simulink model "doublePendulumIMU"  (R2024b)
settings: Solver=VariableStepAuto  StartTime=0.0  StopTime=10.0  MaxStep=0.01  RelTol=1e-3  AbsTol=1e-3  EnableMultiTasking=on
undefined symbols (not defined in the file or in its folder): fractalcoef, X, Y, Z
libraries: nesl_utility x27, sm_lib x11, mspsensorlib x8, matrix_library x2
settings Model: DataDictionary=simData.sldd  Creator=The MathWorks, Inc.  LastModifiedBy=jfing
settings SolverCC: AutoScaleAbsTol=off  AlgebraicLoopSolver=TrustRegion  MaxZcPerStep=1
settings DataIOCC: LimitDataPoints=on  MaxDataPoints=10000
settings OptimizationCC: ReuseModelBlockBuffer=off  LifeSpan=inf
settings DebuggingCC: UnconnectedInputMsg=warning  UnconnectedOutputMsg=warning  UnconnectedLineMsg=warning  AllowSymbolicDim=off  SFUnexpectedBacktrackingDiag=warning  SFNoUnconditionalDefaultTransitionDiag=warning  SFExecutionAtInitializationDiag=none  ArithmeticOperatorsInVariantConditions=warning
settings HardwareCC: ProdHWDeviceType=AMD->x86-64 (Windows64)
settings ModelReferenceCC: EnableRefExpFcnMdlSchedulingChecks=on  EnableParallelModelReferenceBuilds=on  ParallelModelReferenceMATLABWorkerInit=Load Top Model
settings SFSimCC: SimUseLocalCustomCode=off  UsePrecompiledLibraries=Avoid  CustomCodeUndefinedFunction=UseInterfaceOnly  SimTargetLang=C++  GPUAcceleration=on  SimGPUMallocThreshold=1000  SimGPUStackLimitPerThread=2048  SimDLTargetLibrary=cudnn
settings RTWCC: RTWUseLocalCustomCode=off  GPUComputeCapability=3.5  DLArmComputeVersion=19.05
settings CodeAppCC: StateflowObjectComments=on
settings GRTTargetCC: TargetLangStandard=C89/C90 (ANSI)
settings ConfigComp: CovMetricSettings=dw  CovSaveCumulativeToWorkspaceVar=on  CovSaveSingleToWorkspaceVar=on  CovExternalEMLEnable=off  CovSFcnEnable=off
settings SimscapeCC: SimscapeLogType=all  SimscapeLogSimulationStatistics=on  SimscapeLogDataHistory=10000

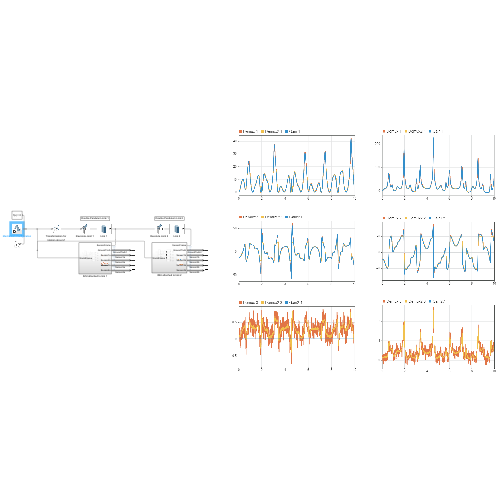
[thumbnail: Simulink's stored preview of the top-level diagram]
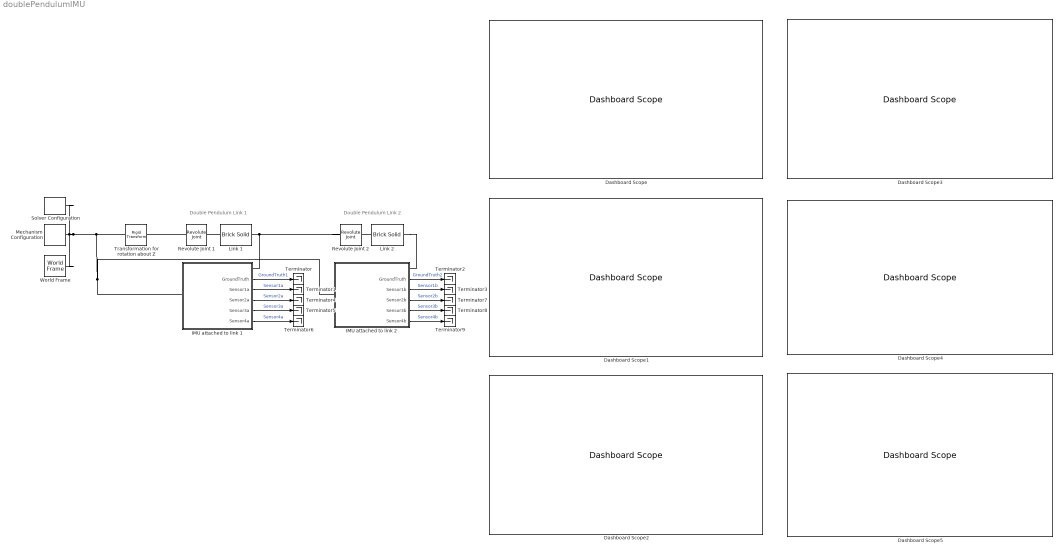
== system doublePendulumIMU ==
  note: Double Pendulum Link 1
  note: Double Pendulum Link 2
  Dashboard Scope{,1..5} (6 alike) : DashboardScope
  IMU attached to link 1 : Subsystem
      settings: PortSchema="{\"entries\":[{\"content\":{\"sides\":[{\"content\":{},\"type\":\"ConnectorPlacement.EquallySpacedRectSide\",\"uuid\":\"7a848249-f78c-431e-84de-981fe01eaf41\"},{\"content\":{\"side\":\"RIGHT\"},\"type\":\"ConnectorPlacement.EquallySpacedRectSide\",\"uuid\":\"a7aca224-ae93-4c7d-a6de-e3d97876bf59\"},{\"content\":{\"connectorIds\":[\"LConn1\"],\"side\":\"TOP\"},\"type\":\"ConnectorPlacement.EquallySpacedRectSide\",\"uuid\":\"e9c2225b-3f07-428c-8b88-abfc95f79ce3\"},{\"content\":{\"connectorIds\":[\"RConn1\",\"Out1\",\"Out2\",\"Out3\",\"Out4\",\"Out5\"],\"side\":\"BOTTOM\"},\"type\":\"ConnectorPlacement.EquallySpacedRectSide\",\"uuid\":\"5c87de37-5620-4b71-be74-049ce4a9ec5b\"}]},\"type\":\"ConnectorPlacement.EquallySpacedConnector\",\"uuid\":\"7bd4f58a-19d1-4168-9367-fe9ef4865104\"}],\"packageUris\":[\"http://schema.mathworks.com/mf0/Connector/R2020b\"],\"version\":\"1.0\"}"
  IMU attached to link 2 : Subsystem
      settings: PortSchema="{\"entries\":[{\"content\":{\"sides\":[{\"content\":{},\"type\":\"ConnectorPlacement.EquallySpacedRectSide\",\"uuid\":\"7a848249-f78c-431e-84de-981fe01eaf41\"},{\"content\":{\"side\":\"RIGHT\"},\"type\":\"ConnectorPlacement.EquallySpacedRectSide\",\"uuid\":\"a7aca224-ae93-4c7d-a6de-e3d97876bf59\"},{\"content\":{\"connectorIds\":[\"LConn1\"],\"side\":\"TOP\"},\"type\":\"ConnectorPlacement.EquallySpacedRectSide\",\"uuid\":\"e9c2225b-3f07-428c-8b88-abfc95f79ce3\"},{\"content\":{\"connectorIds\":[\"RConn1\",\"Out1\",\"Out2\",\"Out3\",\"Out4\",\"Out5\"],\"side\":\"BOTTOM\"},\"type\":\"ConnectorPlacement.EquallySpacedRectSide\",\"uuid\":\"5c87de37-5620-4b71-be74-049ce4a9ec5b\"}]},\"type\":\"ConnectorPlacement.EquallySpacedConnector\",\"uuid\":\"7bd4f58a-19d1-4168-9367-fe9ef4865104\"}],\"packageUris\":[\"http://schema.mathworks.com/mf0/Connector/R2020b\"],\"version\":\"1.0\"}"
  Link 1 : sm_lib/Body Elements/Brick Solid  BrickDimensions=[1 0.1 0.1]  BrickDimensionsUnits=m  ExportEntireGeometry=off  InertiaType=CalculateFromGeometry  BasedOnType=Density  Density=1000  DensityUnits=kg/m^3  Mass=1  MassUnits=kg  CenterOfMass=[0 0 0]  CenterOfMassUnits=m  MomentsOfInertia=[1 1 1]  MomentsOfInertiaUnits=kg*m^2  ProductsOfInertia=[0 0 0]  ProductsOfInertiaUnits=kg*m^2  GraphicType=FromGeometry  MarkerShape=Sphere  MarkerSize=10  GraphicVisPropType=SimpleVisualProperties  GraphicDiffuseColor=[0.5 0.5 0.5]  GraphicOpacity=1.0  GraphicSpecularColor=[0.5 0.5 0.5 1.0]  GraphicAmbientColor=[0.15 0.15 0.15 1.0]  GraphicEmissiveColor=[0.0 0.0 0.0 1.0]  GraphicShininess=75  DoExposeReferenceFrame=off  SerializedFrames=<Frames><Frame><Id>Frame1</Id><Value><Name>F1</Name><Origin><Source>GeometricFeature</Source><FeatureName>-x surface</FeatureName></Origin><PrimaryAxis><DefinedDirection>+Z</DefinedDirection><Source>ReferenceFrame</Source><SourceDirection>+Z</SourceDirection><FeatureName></FeatureName></PrimaryAxis><SecondaryAxis><DefinedDirection>+X</DefinedDirection><Source>ReferenceFrame</Source><SourceDirection>+X</SourceDirection><FeatureName></FeatureName></SecondaryAxis></Value></Frame><Frame><Id>Frame2</Id><Value><Name>F2</Name><Origin><Source>GeometricFeature</Source><FeatureName>+x surface</FeatureName></Origin><PrimaryAxis><DefinedDirection>+Z</DefinedDirection><Source>ReferenceFrame</Source><SourceDirection>+Z</SourceDirection><FeatureName></FeatureName></PrimaryAxis><SecondaryAxis><DefinedDirection>+X</DefinedDirection><Source>ReferenceFrame</Source><SourceDirection>+X</SourceDirection><FeatureName></FeatureName></SecondaryAxis></Value></Frame></Frames>
  Link 2 : sm_lib/Body Elements/Brick Solid  BrickDimensions=[1 0.1 0.1]  BrickDimensionsUnits=m  ExportEntireGeometry=off  InertiaType=CalculateFromGeometry  BasedOnType=Density  Density=1000  DensityUnits=kg/m^3  Mass=1  MassUnits=kg  CenterOfMass=[0 0 0]  CenterOfMassUnits=m  MomentsOfInertia=[1 1 1]  MomentsOfInertiaUnits=kg*m^2  ProductsOfInertia=[0 0 0]  ProductsOfInertiaUnits=kg*m^2  GraphicType=FromGeometry  MarkerShape=Sphere  MarkerSize=10  GraphicVisPropType=SimpleVisualProperties  GraphicDiffuseColor=[0.5 0.5 0.5]  GraphicOpacity=1.0  GraphicSpecularColor=[0.5 0.5 0.5 1.0]  GraphicAmbientColor=[0.15 0.15 0.15 1.0]  GraphicEmissiveColor=[0.0 0.0 0.0 1.0]  GraphicShininess=75  DoExposeReferenceFrame=off  SerializedFrames=<Frames><Frame><Id>Frame1</Id><Value><Name>F1</Name><Origin><Source>GeometricFeature</Source><FeatureName>-x surface</FeatureName></Origin><PrimaryAxis><DefinedDirection>+Z</DefinedDirection><Source>ReferenceFrame</Source><SourceDirection>+Z</SourceDirection><FeatureName></FeatureName></PrimaryAxis><SecondaryAxis><DefinedDirection>+X</DefinedDirection><Source>ReferenceFrame</Source><SourceDirection>+X</SourceDirection><FeatureName></FeatureName></SecondaryAxis></Value></Frame><Frame><Id>Frame2</Id><Value><Name>F2</Name><Origin><Source>GeometricFeature</Source><FeatureName>+x surface</FeatureName></Origin><PrimaryAxis><DefinedDirection>+Z</DefinedDirection><Source>ReferenceFrame</Source><SourceDirection>+Z</SourceDirection><FeatureName></FeatureName></PrimaryAxis><SecondaryAxis><DefinedDirection>+X</DefinedDirection><Source>ReferenceFrame</Source><SourceDirection>+X</SourceDirection><FeatureName></FeatureName></SecondaryAxis></Value></Frame></Frames>
  Mechanism Configuration : sm_lib/Utilities/Mechanism Configuration  UniformGravity=Constant  GravityVector=[0 0 -9.80665]  GravityVectorUnits=m/s^2  LinearizationDelta=0.001  JointModeTransitionNonlinearIterations=2
  Revolute Joint 1 : sm_lib/Joints/Revolute Joint  JointMode=Normal  CompositeWrenchDir=FollowerOnBase  CompositeWrenchFrame=BaseFrame  SenseConstraintForce=off  SenseConstraintTorque=off  SenseTotalForce=off  SenseTotalTorque=off  PositionTargetSpecify=off  PositionTargetPriority=High  PositionTargetValue=0  PositionTargetValueUnits=deg  VelocityTargetSpecify=off  VelocityTargetPriority=High  VelocityTargetValue=0  VelocityTargetValueUnits=deg/s  EquilibriumPosition=0  EquilibriumPositionUnits=deg  SpringStiffness=0  SpringStiffnessUnits=N*m/deg  DampingCoefficient=0  DampingCoefficientUnits=N*m/(deg/s)  LowerLimitSpecify=off  LowerLimitBound=-90  LowerLimitBoundUnits=deg  LowerLimitStiffness=1e4  LowerLimitStiffnessUnits=N*m/deg  LowerLimitDamping=10  LowerLimitDampingUnits=N*m/(deg/s)  LowerLimitTransitionRegionWidth=0.1  LowerLimitTransitionRegionWidthUnits=deg  UpperLimitSpecify=off  UpperLimitBound=90  UpperLimitBoundUnits=deg  UpperLimitStiffness=1e4  UpperLimitStiffnessUnits=N*m/deg  UpperLimitDamping=10  UpperLimitDampingUnits=N*m/(deg/s)  UpperLimitTransitionRegionWidth=0.1  UpperLimitTransitionRegionWidthUnits=deg  TorqueActuationMode=NoTorque  MotionActuationMode=ComputedMotion  SensePosition=off  SenseVelocity=off  SenseAcceleration=off  SenseTorqueForce=off  SenseLowerLimitTorqueForce=off  SenseUpperLimitTorqueForce=off
  Revolute Joint 2 : sm_lib/Joints/Revolute Joint  JointMode=Normal  CompositeWrenchDir=FollowerOnBase  CompositeWrenchFrame=BaseFrame  SenseConstraintForce=off  SenseConstraintTorque=off  SenseTotalForce=off  SenseTotalTorque=off  PositionTargetSpecify=off  PositionTargetPriority=High  PositionTargetValue=0  PositionTargetValueUnits=deg  VelocityTargetSpecify=off  VelocityTargetPriority=High  VelocityTargetValue=0  VelocityTargetValueUnits=deg/s  EquilibriumPosition=0  EquilibriumPositionUnits=deg  SpringStiffness=0  SpringStiffnessUnits=N*m/deg  DampingCoefficient=0  DampingCoefficientUnits=N*m/(deg/s)  LowerLimitSpecify=off  LowerLimitBound=-90  LowerLimitBoundUnits=deg  LowerLimitStiffness=1e4  LowerLimitStiffnessUnits=N*m/deg  LowerLimitDamping=10  LowerLimitDampingUnits=N*m/(deg/s)  LowerLimitTransitionRegionWidth=0.1  LowerLimitTransitionRegionWidthUnits=deg  UpperLimitSpecify=off  UpperLimitBound=90  UpperLimitBoundUnits=deg  UpperLimitStiffness=1e4  UpperLimitStiffnessUnits=N*m/deg  UpperLimitDamping=10  UpperLimitDampingUnits=N*m/(deg/s)  UpperLimitTransitionRegionWidth=0.1  UpperLimitTransitionRegionWidthUnits=deg  TorqueActuationMode=NoTorque  MotionActuationMode=ComputedMotion  SensePosition=off  SenseVelocity=off  SenseAcceleration=off  SenseTorqueForce=off  SenseLowerLimitTorqueForce=off  SenseUpperLimitTorqueForce=off
  Solver Configuration : nesl_utility/Solver Configuration  PhysicalDomain=network_engine_domain  SubClassName=solver  LeftPortType=input  RightPortType=generic  Tones=[]  Harmonics=[]  SimulateNoise=off  Profile=off  UseLocalSampling=off  EnableSwitchedLinearOptims=on  FrequencyDomain=off  UseCCode=off  RelTol=0.001  AbsTol=1e-06  MinStep=1e-09  ToWorkspace=off  RevertToSquareIcSolve=off  NumHomotopyIterations=100  PhasorMode=off  PhasorModeNumHarmonics=1  ConsistencySolver=NEWTON_XTOL_AFTER_FTOL  IndexReductionMethod=DerivativeReplacement  DoDC=off  ResidualTolerance=1e-09  ConsistencyTolSource=GLOBAL  ConsistencyAbsTol=0.001  ConsistencyRelTol=0.001  ConsistencyTolFactor=0.001  UseLocalSolver=off  LocalSolverChoice=NE_BACKWARD_EULER_ADVANCER  ResolveIndetEquations=on  FunctionEvalNumThread=1  LocalSolverSampleTime=0.001  DoFixedCost=off  MaxNonlinIter=3  MaxModeIter=2  ComputeImpulses=off  ImpulseIterations=2  LinearAlgebra=Sparse  LinearAlgebraNumThread=0  EquationFormulation=NE_TIME_EF  DelaysMemoryBudget=1024  AutomaticFiltering=on  FilteringTimeConstant=0.001  PartitionStorageMethod=AS_NEEDED  PartitionMemoryBudget=1024  PartitionMethod=FAST  MultibodyUseLocalSolver=off  MultibodyLocalSolverChoice=ODE1  MultibodyLocalSolverSampleTime=0.001
  Terminator{,1..9} (10 alike) : Terminator
  Transformation for rotation about Z : sm_lib/Frames and Transforms/Rigid Transform  RotationMethod=StandardAxis  FollAlignAxisA=+X  BaseAlignAxisA=+Y  FollAlignAxisB=+Y  BaseAlignAxisB=+Z  RotationStandardAxis=-X  RotationAngle=90  RotationAngleUnits=deg  RotationArbitraryAxis=[0 0 1]  RotationSequenceAxes=FollowerAxes  RotationSequence=XYX  RotationSequenceAngles=[0 0 0]  RotationSequenceAnglesUnits=deg  RotationMatrix=[1 0 0; 0 1 0; 0 0 1]  Quaternion=[1 0 0 0]  TranslationMethod=None  TranslationCartesianOffset=[0 0 0]  TranslationCartesianOffsetUnits=m  TranslationStandardAxis=+Z  TranslationStandardOffset=0  TranslationStandardOffsetUnits=m  TranslationROffset=0  TranslationROffsetUnits=m  TranslationThetaOffset=0  TranslationThetaOffsetUnits=deg  TranslationZOffset=0  TranslationZOffsetUnits=m
  World Frame : sm_lib/Frames and Transforms/World Frame
  wires:
  IMU attached to link 1/1(GroundTruth) -> Terminator/1  "GroundTruth1"
  IMU attached to link 1/2(Sensor1a) -> Terminator1/1  "Sensor1a"
  IMU attached to link 2/2(Sensor1b) -> Terminator3/1  "Sensor1b"
  IMU attached to link 2/1(GroundTruth) -> Terminator2/1  "GroundTruth2"
  IMU attached to link 1/3(Sensor2a) -> Terminator4/1  "Sensor2a"
  IMU attached to link 1/4(Sensor3a) -> Terminator5/1  "Sensor3a"
  IMU attached to link 1/5(Sensor4a) -> Terminator6/1  "Sensor4a"
  IMU attached to link 2/3(Sensor2b) -> Terminator7/1  "Sensor2b"
  IMU attached to link 2/4(Sensor3b) -> Terminator8/1  "Sensor3b"
  IMU attached to link 2/5(Sensor4b) -> Terminator9/1  "Sensor4b"
  connections:
  Link 1/LConn1 -- Revolute Joint 1/RConn1
  Revolute Joint 1/LConn1 -- Transformation for rotation about Z/RConn1
  IMU attached to link 1/RConn1 -- Revolute Joint 2/LConn1 -- Link 1/RConn1
  Link 2/LConn1 -- Revolute Joint 2/RConn1
  Link 2/RConn1 -- IMU attached to link 2/RConn1
  IMU attached to link 1/LConn1 -- IMU attached to link 2/LConn1 -- Transformation for rotation about Z/LConn1 -- World Frame/RConn1 -- Solver Configuration/RConn1 -- Mechanism Configuration/RConn1

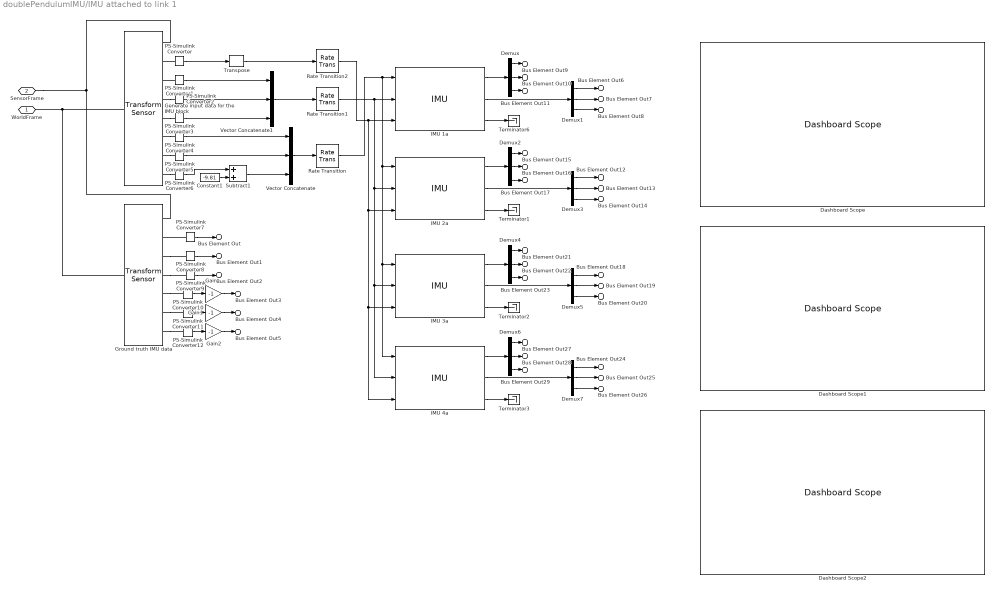
== system doublePendulumIMU/IMU attached to link 1 ==
  Constant1 : Constant  Value=-9.81
  Dashboard Scope : DashboardScope
  Dashboard Scope1 : DashboardScope
  Dashboard Scope2 : DashboardScope
  Demux{,1..7} (8 alike) : Demux  Outputs=3
  Gain : Gain  Gain=-1
  Gain1 : Gain  Gain=-1
  Gain2 : Gain  Gain=-1
  Generate input data for the IMU block : sm_lib/Frames and Transforms/Transform Sensor  MeasurementFrame=World  RotationSequence=XYX  SenseAngle=off  SenseAxis=off  SenseQ=on  SenseR=off  SenseRotationSequence=off  SenseOmegaX=on  SenseOmegaY=on  SenseOmegaZ=on  SenseOmega=off  SenseQDot=off  SenseRDot=off  SenseRotationSequenceDot=off  SenseAlphaX=off  SenseAlphaY=off  SenseAlphaZ=off  SenseAlpha=off  SenseQDDot=off  SenseRDDot=off  SenseX=off  SenseY=off  SenseZ=off  SenseXYZ=off  SenseRad=off  SenseAzim=off  SenseDist=off  SenseInc=off  SenseXDot=off  SenseYDot=off  SenseZDot=off  SenseXYZDot=off  SenseRadDot=off  SenseAzimDot=off  SenseDistDot=off  SenseIncDot=off  SenseXDDot=on  SenseYDDot=on  SenseZDDot=on  SenseXYZDDot=off  SenseRadDDot=off  SenseAzimDDot=off  SenseDistDDot=off  SenseIncDDot=off
  Ground truth IMU data : sm_lib/Frames and Transforms/Transform Sensor  MeasurementFrame=NonRotatingFollower  RotationSequence=XYX  SenseAngle=off  SenseAxis=off  SenseQ=off  SenseR=off  SenseRotationSequence=off  SenseOmegaX=on  SenseOmegaY=on  SenseOmegaZ=on  SenseOmega=off  SenseQDot=off  SenseRDot=off  SenseRotationSequenceDot=off  SenseAlphaX=off  SenseAlphaY=off  SenseAlphaZ=off  SenseAlpha=off  SenseQDDot=off  SenseRDDot=off  SenseX=off  SenseY=off  SenseZ=off  SenseXYZ=off  SenseRad=off  SenseAzim=off  SenseDist=off  SenseInc=off  SenseXDot=off  SenseYDot=off  SenseZDot=off  SenseXYZDot=off  SenseRadDot=off  SenseAzimDot=off  SenseDistDot=off  SenseIncDot=off  SenseXDDot=on  SenseYDDot=on  SenseZDDot=on  SenseXYZDDot=off  SenseRadDDot=off  SenseAzimDDot=off  SenseDistDDot=off  SenseIncDDot=off
  IMU 1a : mspsensorlib/IMU  DispRefFrame=ENU  TemperaturePort=off  Temperature=25  MagneticFieldPort=off  MagneticFieldNED=[ 27.5550, -2.4169, -16.0849 ]  MagneticFieldENU=[ -2.4169, 27.5550, 16.0849 ]  SeedDouble=67  SimulateUsing=Interpreted execution  AccelParamsMeasurementRange=156.9064  AccelParamsResolution=4.9791e-05  AccelParamsConstantBias=0.196133  AccelParamsAxesMisalignment=1  AccelParamsNoiseDensity=0.00063743225  AccelParamsBiasInstability=0.15691  AccelParamsBiasInstabilityNumerator=fractalcoef().Numerator  AccelParamsBiasInstabilityDenominator=fractalcoef().Denominator  AccelParamsRandomWalk=[ 0, 0, 0 ]  AccelParamsNoiseType=double-sided  AccelParamsTemperatureBias=0.0014709975  AccelParamsTemperatureScaleFactor=0.005  GyroParamsMeasurementRange=34.9066  GyroParamsResolution=3.4936  GyroParamsConstantBias=0.00872664625997165  GyroParamsAxesMisalignment=1.25  GyroParamsAccelerationBias=[ 0, 0, 0 ]  GyroParamsNoiseDensity=0.000488692190558412  GyroParamsBiasInstability=0.034907  GyroParamsBiasInstabilityNumerator=fractalcoef().Numerator  GyroParamsBiasInstabilityDenominator=fractalcoef().Denominator  GyroParamsRandomWalk=[ 0, 0, 0 ]  GyroParamsNoiseType=double-sided  GyroParamsTemperatureBias=8.72664625997165e-05  GyroParamsTemperatureScaleFactor=0.005  MagParamsMeasurementRange=Inf  MagParamsResolution=0  MagParamsConstantBias=[ 0, 0, 0 ]  MagParamsAxesMisalignment=[ 100, 0, 0; 0, 100, 0; 0, 0, 100 ]  MagParamsNoiseDensity=[ 0, 0, 0 ]  MagParamsBiasInstability=[ 0, 0, 0 ]  MagParamsBiasInstabilityNumerator=fractalcoef().Numerator  MagParamsBiasInstabilityDenominator=fractalcoef().Denominator  MagParamsRandomWalk=[ 0, 0, 0 ]  MagParamsNoiseType=double-sided  MagParamsTemperatureBias=[ 0, 0, 0 ]  MagParamsTemperatureScaleFactor=[ 0, 0, 0 ]
  IMU 2a : mspsensorlib/IMU  DispRefFrame=ENU  TemperaturePort=off  Temperature=25  MagneticFieldPort=off  MagneticFieldNED=[ 27.5550, -2.4169, -16.0849 ]  MagneticFieldENU=[ -2.4169, 27.5550, 16.0849 ]  SeedDouble=67  SimulateUsing=Interpreted execution  AccelParamsMeasurementRange=19.6133  AccelParamsResolution=6.2239e-06  AccelParamsConstantBias=0.196133  AccelParamsAxesMisalignment=1  AccelParamsNoiseDensity=0.00063743225  AccelParamsBiasInstability=0.019613  AccelParamsBiasInstabilityNumerator=fractalcoef().Numerator  AccelParamsBiasInstabilityDenominator=fractalcoef().Denominator  AccelParamsRandomWalk=[ 0, 0, 0 ]  AccelParamsNoiseType=double-sided  AccelParamsTemperatureBias=0.0014709975  AccelParamsTemperatureScaleFactor=0.005  GyroParamsMeasurementRange=4.3633  GyroParamsResolution=0.43737  GyroParamsConstantBias=0.00872664625997165  GyroParamsAxesMisalignment=1.25  GyroParamsAccelerationBias=[ 0, 0, 0 ]  GyroParamsNoiseDensity=0.000488692190558412  GyroParamsBiasInstability=0.0043633  GyroParamsBiasInstabilityNumerator=fractalcoef().Numerator  GyroParamsBiasInstabilityDenominator=fractalcoef().Denominator  GyroParamsRandomWalk=[ 0, 0, 0 ]  GyroParamsNoiseType=double-sided  GyroParamsTemperatureBias=8.72664625997165e-05  GyroParamsTemperatureScaleFactor=0.005  MagParamsMeasurementRange=Inf  MagParamsResolution=0  MagParamsConstantBias=[ 0, 0, 0 ]  MagParamsAxesMisalignment=[ 100, 0, 0; 0, 100, 0; 0, 0, 100 ]  MagParamsNoiseDensity=[ 0, 0, 0 ]  MagParamsBiasInstability=[ 0, 0, 0 ]  MagParamsBiasInstabilityNumerator=fractalcoef().Numerator  MagParamsBiasInstabilityDenominator=fractalcoef().Denominator  MagParamsRandomWalk=[ 0, 0, 0 ]  MagParamsNoiseType=double-sided  MagParamsTemperatureBias=[ 0, 0, 0 ]  MagParamsTemperatureScaleFactor=[ 0, 0, 0 ]
  IMU 3a : mspsensorlib/IMU  DispRefFrame=ENU  TemperaturePort=off  Temperature=25  MagneticFieldPort=off  MagneticFieldNED=[ 27.5550, -2.4169, -16.0849 ]  MagneticFieldENU=[ -2.4169, 27.5550, 16.0849 ]  SeedDouble=67  SimulateUsing=Interpreted execution  AccelParamsMeasurementRange=156.9064  AccelParamsResolution=4.9791e-05  AccelParamsConstantBias=0.196133  AccelParamsAxesMisalignment=1  AccelParamsNoiseDensity=0.00063743225  AccelParamsBiasInstability=0.15691  AccelParamsBiasInstabilityNumerator=fractalcoef().Numerator  AccelParamsBiasInstabilityDenominator=fractalcoef().Denominator  AccelParamsRandomWalk=[ 0, 0, 0 ]  AccelParamsNoiseType=double-sided  AccelParamsTemperatureBias=0.0014709975  AccelParamsTemperatureScaleFactor=0.005  GyroParamsMeasurementRange=34.9066  GyroParamsResolution=3.4936  GyroParamsConstantBias=0.00872664625997165  GyroParamsAxesMisalignment=1.25  GyroParamsAccelerationBias=[ 0, 0, 0 ]  GyroParamsNoiseDensity=0.000488692190558412  GyroParamsBiasInstability=0.034907  GyroParamsBiasInstabilityNumerator=fractalcoef().Numerator  GyroParamsBiasInstabilityDenominator=fractalcoef().Denominator  GyroParamsRandomWalk=[ 0, 0, 0 ]  GyroParamsNoiseType=double-sided  GyroParamsTemperatureBias=8.72664625997165e-05  GyroParamsTemperatureScaleFactor=0.005  MagParamsMeasurementRange=Inf  MagParamsResolution=0  MagParamsConstantBias=[ 0, 0, 0 ]  MagParamsAxesMisalignment=[ 100, 0, 0; 0, 100, 0; 0, 0, 100 ]  MagParamsNoiseDensity=[ 0, 0, 0 ]  MagParamsBiasInstability=[ 0, 0, 0 ]  MagParamsBiasInstabilityNumerator=fractalcoef().Numerator  MagParamsBiasInstabilityDenominator=fractalcoef().Denominator  MagParamsRandomWalk=[ 0, 0, 0 ]  MagParamsNoiseType=double-sided  MagParamsTemperatureBias=[ 0, 0, 0 ]  MagParamsTemperatureScaleFactor=[ 0, 0, 0 ]
  IMU 4a : mspsensorlib/IMU  DispRefFrame=ENU  TemperaturePort=off  Temperature=25  MagneticFieldPort=off  MagneticFieldNED=[ 27.5550, -2.4169, -16.0849 ]  MagneticFieldENU=[ -2.4169, 27.5550, 16.0849 ]  SeedDouble=67  SimulateUsing=Interpreted execution  AccelParamsMeasurementRange=19.6133  AccelParamsResolution=6.2239e-06  AccelParamsConstantBias=0.196133  AccelParamsAxesMisalignment=1  AccelParamsNoiseDensity=0.00063743225  AccelParamsBiasInstability=0.019613  AccelParamsBiasInstabilityNumerator=fractalcoef().Numerator  AccelParamsBiasInstabilityDenominator=fractalcoef().Denominator  AccelParamsRandomWalk=[ 0, 0, 0 ]  AccelParamsNoiseType=double-sided  AccelParamsTemperatureBias=0.0014709975  AccelParamsTemperatureScaleFactor=0.005  GyroParamsMeasurementRange=4.3633  GyroParamsResolution=0.43737  GyroParamsConstantBias=0.00872664625997165  GyroParamsAxesMisalignment=1.25  GyroParamsAccelerationBias=[ 0, 0, 0 ]  GyroParamsNoiseDensity=0.000488692190558412  GyroParamsBiasInstability=0.0043633  GyroParamsBiasInstabilityNumerator=fractalcoef().Numerator  GyroParamsBiasInstabilityDenominator=fractalcoef().Denominator  GyroParamsRandomWalk=[ 0, 0, 0 ]  GyroParamsNoiseType=double-sided  GyroParamsTemperatureBias=8.72664625997165e-05  GyroParamsTemperatureScaleFactor=0.005  MagParamsMeasurementRange=Inf  MagParamsResolution=0  MagParamsConstantBias=[ 0, 0, 0 ]  MagParamsAxesMisalignment=[ 100, 0, 0; 0, 100, 0; 0, 0, 100 ]  MagParamsNoiseDensity=[ 0, 0, 0 ]  MagParamsBiasInstability=[ 0, 0, 0 ]  MagParamsBiasInstabilityNumerator=fractalcoef().Numerator  MagParamsBiasInstabilityDenominator=fractalcoef().Denominator  MagParamsRandomWalk=[ 0, 0, 0 ]  MagParamsNoiseType=double-sided  MagParamsTemperatureBias=[ 0, 0, 0 ]  MagParamsTemperatureScaleFactor=[ 0, 0, 0 ]
  PS-Simulink Converter : nesl_utility/PS-Simulink Converter  PhysicalDomain=network_engine_domain  SubClassName=ps_output  LeftPortType=input  RightPortType=output  PseudoPeriodic=off  Frequencies=[]  VectorFormat=inherit  Unit=rad  AffineConversion=off
  PS-Simulink Converter{1..3,7..9} (6 alike) : nesl_utility/PS-Simulink Converter  PhysicalDomain=network_engine_domain  SubClassName=ps_output  LeftPortType=input  RightPortType=output  PseudoPeriodic=off  Frequencies=[]  VectorFormat=inherit  Unit=rad/s  AffineConversion=off
  PS-Simulink Converter{4..6,10..12} (6 alike) : nesl_utility/PS-Simulink Converter  PhysicalDomain=network_engine_domain  SubClassName=ps_output  LeftPortType=input  RightPortType=output  PseudoPeriodic=off  Frequencies=[]  VectorFormat=inherit  Unit=m/s^2  AffineConversion=off
  Rate Transition : RateTransition  OutPortSampleTime=Fs_time
  Rate Transition1 : RateTransition  OutPortSampleTime=Fs_time
  Rate Transition2 : RateTransition  OutPortSampleTime=Fs_time
  Subtract1 : Sum
  Terminator{1..3,6} (4 alike) : Terminator
  Transpose : matrix_library/Transpose
  Vector Concatenate : Concatenate  NumInputs=3  Mode=Multidimensional array  ConcatenateDimension=2
  Vector Concatenate1 : Concatenate  NumInputs=3  Mode=Multidimensional array  ConcatenateDimension=2
  WorldFrame : PMIOPort  Side=Left
  SensorFrame : PMIOPort  Port=2  Side=Right
  Bus Element Out3 : Outport  PortName=GroundTruth  Element=ax
  Bus Element Out4 : Outport  PortName=GroundTruth  Element=ay
  Bus Element Out5 : Outport  PortName=GroundTruth  Element=az
  Bus Element Out : Outport  PortName=GroundTruth  Element=wx
  Bus Element Out1 : Outport  PortName=GroundTruth  Element=wy
  Bus Element Out2 : Outport  PortName=GroundTruth  Element=wz
  Bus Element Out6 : Outport  Port=2  PortName=Sensor1a  Element=wx
  Bus Element Out7 : Outport  Port=2  PortName=Sensor1a  Element=wy
  Bus Element Out8 : Outport  Port=2  PortName=Sensor1a  Element=wz
  Bus Element Out9 : Outport  Port=2  PortName=Sensor1a  Element=ax
  Bus Element Out10 : Outport  Port=2  PortName=Sensor1a  Element=ay
  Bus Element Out11 : Outport  Port=2  PortName=Sensor1a  Element=az
  Bus Element Out12 : Outport  Port=3  PortName=Sensor2a  Element=wx
  Bus Element Out13 : Outport  Port=3  PortName=Sensor2a  Element=wy
  Bus Element Out14 : Outport  Port=3  PortName=Sensor2a  Element=wz
  Bus Element Out15 : Outport  Port=3  PortName=Sensor2a  Element=ax
  Bus Element Out16 : Outport  Port=3  PortName=Sensor2a  Element=ay
  Bus Element Out17 : Outport  Port=3  PortName=Sensor2a  Element=az
  Bus Element Out18 : Outport  Port=4  PortName=Sensor3a  Element=wx
  Bus Element Out19 : Outport  Port=4  PortName=Sensor3a  Element=wy
  Bus Element Out20 : Outport  Port=4  PortName=Sensor3a  Element=wz
  Bus Element Out21 : Outport  Port=4  PortName=Sensor3a  Element=ax
  Bus Element Out22 : Outport  Port=4  PortName=Sensor3a  Element=ay
  Bus Element Out23 : Outport  Port=4  PortName=Sensor3a  Element=az
  Bus Element Out24 : Outport  Port=5  PortName=Sensor4a  Element=wx
  Bus Element Out25 : Outport  Port=5  PortName=Sensor4a  Element=wy
  Bus Element Out26 : Outport  Port=5  PortName=Sensor4a  Element=wz
  Bus Element Out27 : Outport  Port=5  PortName=Sensor4a  Element=ax
  Bus Element Out28 : Outport  Port=5  PortName=Sensor4a  Element=ay
  Bus Element Out29 : Outport  Port=5  PortName=Sensor4a  Element=az
  wires:
  PS-Simulink Converter4/1 -> Vector Concatenate/1
  IMU 1a/3 -> Terminator6/1
  PS-Simulink Converter6/1 -> Subtract1/1
  PS-Simulink Converter3/1 -> Vector Concatenate1/3
  PS-Simulink Converter1/1 -> Vector Concatenate1/1
  PS-Simulink Converter2/1 -> Vector Concatenate1/2
  Vector Concatenate1/1 -> Rate Transition1/1
  Rate Transition/1 -> IMU 4a/1, IMU 3a/1, IMU 2a/1, IMU 1a/1
  PS-Simulink Converter12/1 -> Gain2/1
  PS-Simulink Converter/1 -> Transpose/1
  PS-Simulink Converter10/1 -> Gain/1
  PS-Simulink Converter5/1 -> Vector Concatenate/2
  Transpose/1 -> Rate Transition2/1
  Demux/3 -> Bus Element Out11/1
  Demux/1 -> Bus Element Out9/1
  IMU 1a/2 -> Demux1/1
  IMU 1a/1 -> Demux/1
  PS-Simulink Converter11/1 -> Gain1/1
  Rate Transition1/1 -> IMU 1a/2, IMU 3a/2, IMU 4a/2, IMU 2a/2
  Vector Concatenate/1 -> Rate Transition/1
  Subtract1/1 -> Vector Concatenate/3
  Demux/2 -> Bus Element Out10/1
  Rate Transition2/1 -> IMU 4a/3, IMU 3a/3, IMU 2a/3, IMU 1a/3
  Constant1/1 -> Subtract1/2
  Demux1/1 -> Bus Element Out6/1
  Demux1/2 -> Bus Element Out7/1
  Demux1/3 -> Bus Element Out8/1
  PS-Simulink Converter7/1 -> Bus Element Out/1
  PS-Simulink Converter8/1 -> Bus Element Out1/1
  PS-Simulink Converter9/1 -> Bus Element Out2/1
  Gain/1 -> Bus Element Out3/1
  Gain1/1 -> Bus Element Out4/1
  Gain2/1 -> Bus Element Out5/1
  IMU 2a/1 -> Demux2/1
  IMU 2a/3 -> Terminator1/1
  Demux2/1 -> Bus Element Out15/1
  Demux3/2 -> Bus Element Out13/1
  Demux3/1 -> Bus Element Out12/1
  IMU 2a/2 -> Demux3/1
  Demux3/3 -> Bus Element Out14/1
  Demux2/2 -> Bus Element Out16/1
  Demux2/3 -> Bus Element Out17/1
  IMU 3a/1 -> Demux4/1
  IMU 3a/3 -> Terminator2/1
  Demux4/1 -> Bus Element Out21/1
  Demux5/2 -> Bus Element Out19/1
  Demux5/1 -> Bus Element Out18/1
  IMU 3a/2 -> Demux5/1
  Demux5/3 -> Bus Element Out20/1
  Demux4/2 -> Bus Element Out22/1
  Demux4/3 -> Bus Element Out23/1
  IMU 4a/1 -> Demux6/1
  IMU 4a/3 -> Terminator3/1
  Demux6/1 -> Bus Element Out27/1
  Demux7/2 -> Bus Element Out25/1
  Demux7/1 -> Bus Element Out24/1
  IMU 4a/2 -> Demux7/1
  Demux7/3 -> Bus Element Out26/1
  Demux6/2 -> Bus Element Out28/1
  Demux6/3 -> Bus Element Out29/1
  connections:
  SensorFrame/RConn1 -- Generate input data for the IMU block/RConn1 -- Ground truth IMU data/RConn1
  PS-Simulink Converter/LConn1 -- Generate input data for the IMU block/RConn2
  Generate input data for the IMU block/RConn5 -- PS-Simulink Converter3/LConn1
  Generate input data for the IMU block/RConn4 -- PS-Simulink Converter2/LConn1
  Generate input data for the IMU block/LConn1 -- Ground truth IMU data/LConn1 -- WorldFrame/RConn1
  Generate input data for the IMU block/RConn8 -- PS-Simulink Converter6/LConn1
  Generate input data for the IMU block/RConn7 -- PS-Simulink Converter5/LConn1
  PS-Simulink Converter1/LConn1 -- Generate input data for the IMU block/RConn3
  Generate input data for the IMU block/RConn6 -- PS-Simulink Converter4/LConn1
  Ground truth IMU data/RConn5 -- PS-Simulink Converter10/LConn1
  Ground truth IMU data/RConn6 -- PS-Simulink Converter11/LConn1
  Ground truth IMU data/RConn7 -- PS-Simulink Converter12/LConn1
  Ground truth IMU data/RConn4 -- PS-Simulink Converter9/LConn1
  PS-Simulink Converter7/LConn1 -- Ground truth IMU data/RConn2
  Ground truth IMU data/RConn3 -- PS-Simulink Converter8/LConn1

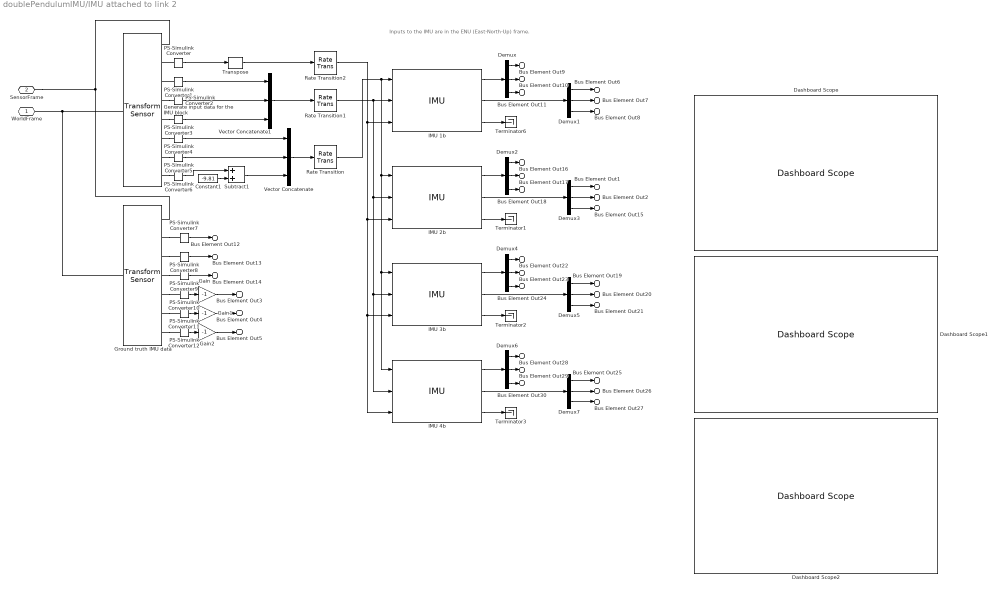
== system doublePendulumIMU/IMU attached to link 2 ==
  note: Inputs to the IMU are in the ENU (East-North-Up) frame.
  Constant1 : Constant  Value=-9.81
  Dashboard Scope : DashboardScope
  Dashboard Scope1 : DashboardScope
  Dashboard Scope2 : DashboardScope
  Demux{,1..7} (8 alike) : Demux  Outputs=3
  Gain : Gain  Gain=-1
  Gain1 : Gain  Gain=-1
  Gain2 : Gain  Gain=-1
  Generate input data for the IMU block : sm_lib/Frames and Transforms/Transform Sensor  MeasurementFrame=World  RotationSequence=XYX  SenseAngle=off  SenseAxis=off  SenseQ=on  SenseR=off  SenseRotationSequence=off  SenseOmegaX=on  SenseOmegaY=on  SenseOmegaZ=on  SenseOmega=off  SenseQDot=off  SenseRDot=off  SenseRotationSequenceDot=off  SenseAlphaX=off  SenseAlphaY=off  SenseAlphaZ=off  SenseAlpha=off  SenseQDDot=off  SenseRDDot=off  SenseX=off  SenseY=off  SenseZ=off  SenseXYZ=off  SenseRad=off  SenseAzim=off  SenseDist=off  SenseInc=off  SenseXDot=off  SenseYDot=off  SenseZDot=off  SenseXYZDot=off  SenseRadDot=off  SenseAzimDot=off  SenseDistDot=off  SenseIncDot=off  SenseXDDot=on  SenseYDDot=on  SenseZDDot=on  SenseXYZDDot=off  SenseRadDDot=off  SenseAzimDDot=off  SenseDistDDot=off  SenseIncDDot=off
  Ground truth IMU data : sm_lib/Frames and Transforms/Transform Sensor  MeasurementFrame=NonRotatingFollower  RotationSequence=XYX  SenseAngle=off  SenseAxis=off  SenseQ=off  SenseR=off  SenseRotationSequence=off  SenseOmegaX=on  SenseOmegaY=on  SenseOmegaZ=on  SenseOmega=off  SenseQDot=off  SenseRDot=off  SenseRotationSequenceDot=off  SenseAlphaX=off  SenseAlphaY=off  SenseAlphaZ=off  SenseAlpha=off  SenseQDDot=off  SenseRDDot=off  SenseX=off  SenseY=off  SenseZ=off  SenseXYZ=off  SenseRad=off  SenseAzim=off  SenseDist=off  SenseInc=off  SenseXDot=off  SenseYDot=off  SenseZDot=off  SenseXYZDot=off  SenseRadDot=off  SenseAzimDot=off  SenseDistDot=off  SenseIncDot=off  SenseXDDot=on  SenseYDDot=on  SenseZDDot=on  SenseXYZDDot=off  SenseRadDDot=off  SenseAzimDDot=off  SenseDistDDot=off  SenseIncDDot=off
  IMU 1b : mspsensorlib/IMU  DispRefFrame=ENU  TemperaturePort=off  Temperature=25  MagneticFieldPort=off  MagneticFieldNED=[ 27.5550, -2.4169, -16.0849 ]  MagneticFieldENU=[ -2.4169, 27.5550, 16.0849 ]  SeedDouble=67  SimulateUsing=Interpreted execution  AccelParamsMeasurementRange=156.9064  AccelParamsResolution=4.9791e-05  AccelParamsConstantBias=0.196133  AccelParamsAxesMisalignment=1  AccelParamsNoiseDensity=0.00063743225  AccelParamsBiasInstability=0.15691  AccelParamsBiasInstabilityNumerator=fractalcoef().Numerator  AccelParamsBiasInstabilityDenominator=fractalcoef().Denominator  AccelParamsRandomWalk=[ 0, 0, 0 ]  AccelParamsNoiseType=double-sided  AccelParamsTemperatureBias=0.0014709975  AccelParamsTemperatureScaleFactor=0.005  GyroParamsMeasurementRange=34.9066  GyroParamsResolution=3.4936  GyroParamsConstantBias=0.00872664625997165  GyroParamsAxesMisalignment=1.25  GyroParamsAccelerationBias=[ 0, 0, 0 ]  GyroParamsNoiseDensity=0.000488692190558412  GyroParamsBiasInstability=0.034907  GyroParamsBiasInstabilityNumerator=fractalcoef().Numerator  GyroParamsBiasInstabilityDenominator=fractalcoef().Denominator  GyroParamsRandomWalk=[ 0, 0, 0 ]  GyroParamsNoiseType=double-sided  GyroParamsTemperatureBias=8.72664625997165e-05  GyroParamsTemperatureScaleFactor=0.005  MagParamsMeasurementRange=Inf  MagParamsResolution=0  MagParamsConstantBias=[ 0, 0, 0 ]  MagParamsAxesMisalignment=[ 100, 0, 0; 0, 100, 0; 0, 0, 100 ]  MagParamsNoiseDensity=[ 0, 0, 0 ]  MagParamsBiasInstability=[ 0, 0, 0 ]  MagParamsBiasInstabilityNumerator=fractalcoef().Numerator  MagParamsBiasInstabilityDenominator=fractalcoef().Denominator  MagParamsRandomWalk=[ 0, 0, 0 ]  MagParamsNoiseType=double-sided  MagParamsTemperatureBias=[ 0, 0, 0 ]  MagParamsTemperatureScaleFactor=[ 0, 0, 0 ]
  IMU 2b : mspsensorlib/IMU  DispRefFrame=ENU  TemperaturePort=off  Temperature=25  MagneticFieldPort=off  MagneticFieldNED=[ 27.5550, -2.4169, -16.0849 ]  MagneticFieldENU=[ -2.4169, 27.5550, 16.0849 ]  SeedDouble=67  SimulateUsing=Interpreted execution  AccelParamsMeasurementRange=19.6133  AccelParamsResolution=6.2239e-06  AccelParamsConstantBias=0.196133  AccelParamsAxesMisalignment=1  AccelParamsNoiseDensity=0.00063743225  AccelParamsBiasInstability=0.019613  AccelParamsBiasInstabilityNumerator=fractalcoef().Numerator  AccelParamsBiasInstabilityDenominator=fractalcoef().Denominator  AccelParamsRandomWalk=[ 0, 0, 0 ]  AccelParamsNoiseType=double-sided  AccelParamsTemperatureBias=0.0014709975  AccelParamsTemperatureScaleFactor=0.005  GyroParamsMeasurementRange=4.3633  GyroParamsResolution=0.43737  GyroParamsConstantBias=0.00872664625997165  GyroParamsAxesMisalignment=1.25  GyroParamsAccelerationBias=[ 0, 0, 0 ]  GyroParamsNoiseDensity=0.000488692190558412  GyroParamsBiasInstability=0.0043633  GyroParamsBiasInstabilityNumerator=fractalcoef().Numerator  GyroParamsBiasInstabilityDenominator=fractalcoef().Denominator  GyroParamsRandomWalk=[ 0, 0, 0 ]  GyroParamsNoiseType=double-sided  GyroParamsTemperatureBias=8.72664625997165e-05  GyroParamsTemperatureScaleFactor=0.005  MagParamsMeasurementRange=Inf  MagParamsResolution=0  MagParamsConstantBias=[ 0, 0, 0 ]  MagParamsAxesMisalignment=[ 100, 0, 0; 0, 100, 0; 0, 0, 100 ]  MagParamsNoiseDensity=[ 0, 0, 0 ]  MagParamsBiasInstability=[ 0, 0, 0 ]  MagParamsBiasInstabilityNumerator=fractalcoef().Numerator  MagParamsBiasInstabilityDenominator=fractalcoef().Denominator  MagParamsRandomWalk=[ 0, 0, 0 ]  MagParamsNoiseType=double-sided  MagParamsTemperatureBias=[ 0, 0, 0 ]  MagParamsTemperatureScaleFactor=[ 0, 0, 0 ]
  IMU 3b : mspsensorlib/IMU  DispRefFrame=ENU  TemperaturePort=off  Temperature=25  MagneticFieldPort=off  MagneticFieldNED=[ 27.5550, -2.4169, -16.0849 ]  MagneticFieldENU=[ -2.4169, 27.5550, 16.0849 ]  SeedDouble=67  SimulateUsing=Interpreted execution  AccelParamsMeasurementRange=156.9064  AccelParamsResolution=4.9791e-05  AccelParamsConstantBias=0.196133  AccelParamsAxesMisalignment=1  AccelParamsNoiseDensity=0.00063743225  AccelParamsBiasInstability=0.15691  AccelParamsBiasInstabilityNumerator=fractalcoef().Numerator  AccelParamsBiasInstabilityDenominator=fractalcoef().Denominator  AccelParamsRandomWalk=[ 0, 0, 0 ]  AccelParamsNoiseType=double-sided  AccelParamsTemperatureBias=0.0014709975  AccelParamsTemperatureScaleFactor=0.005  GyroParamsMeasurementRange=34.9066  GyroParamsResolution=3.4936  GyroParamsConstantBias=0.00872664625997165  GyroParamsAxesMisalignment=1.25  GyroParamsAccelerationBias=[ 0, 0, 0 ]  GyroParamsNoiseDensity=0.000488692190558412  GyroParamsBiasInstability=0.034907  GyroParamsBiasInstabilityNumerator=fractalcoef().Numerator  GyroParamsBiasInstabilityDenominator=fractalcoef().Denominator  GyroParamsRandomWalk=[ 0, 0, 0 ]  GyroParamsNoiseType=double-sided  GyroParamsTemperatureBias=8.72664625997165e-05  GyroParamsTemperatureScaleFactor=0.005  MagParamsMeasurementRange=Inf  MagParamsResolution=0  MagParamsConstantBias=[ 0, 0, 0 ]  MagParamsAxesMisalignment=[ 100, 0, 0; 0, 100, 0; 0, 0, 100 ]  MagParamsNoiseDensity=[ 0, 0, 0 ]  MagParamsBiasInstability=[ 0, 0, 0 ]  MagParamsBiasInstabilityNumerator=fractalcoef().Numerator  MagParamsBiasInstabilityDenominator=fractalcoef().Denominator  MagParamsRandomWalk=[ 0, 0, 0 ]  MagParamsNoiseType=double-sided  MagParamsTemperatureBias=[ 0, 0, 0 ]  MagParamsTemperatureScaleFactor=[ 0, 0, 0 ]
  IMU 4b : mspsensorlib/IMU  DispRefFrame=ENU  TemperaturePort=off  Temperature=25  MagneticFieldPort=off  MagneticFieldNED=[ 27.5550, -2.4169, -16.0849 ]  MagneticFieldENU=[ -2.4169, 27.5550, 16.0849 ]  SeedDouble=67  SimulateUsing=Interpreted execution  AccelParamsMeasurementRange=19.6133  AccelParamsResolution=6.2239e-06  AccelParamsConstantBias=0.196133  AccelParamsAxesMisalignment=1  AccelParamsNoiseDensity=0.00063743225  AccelParamsBiasInstability=0.019613  AccelParamsBiasInstabilityNumerator=fractalcoef().Numerator  AccelParamsBiasInstabilityDenominator=fractalcoef().Denominator  AccelParamsRandomWalk=[ 0, 0, 0 ]  AccelParamsNoiseType=double-sided  AccelParamsTemperatureBias=0.0014709975  AccelParamsTemperatureScaleFactor=0.005  GyroParamsMeasurementRange=4.3633  GyroParamsResolution=0.43737  GyroParamsConstantBias=0.00872664625997165  GyroParamsAxesMisalignment=1.25  GyroParamsAccelerationBias=[ 0, 0, 0 ]  GyroParamsNoiseDensity=0.000488692190558412  GyroParamsBiasInstability=0.0043633  GyroParamsBiasInstabilityNumerator=fractalcoef().Numerator  GyroParamsBiasInstabilityDenominator=fractalcoef().Denominator  GyroParamsRandomWalk=[ 0, 0, 0 ]  GyroParamsNoiseType=double-sided  GyroParamsTemperatureBias=8.72664625997165e-05  GyroParamsTemperatureScaleFactor=0.005  MagParamsMeasurementRange=Inf  MagParamsResolution=0  MagParamsConstantBias=[ 0, 0, 0 ]  MagParamsAxesMisalignment=[ 100, 0, 0; 0, 100, 0; 0, 0, 100 ]  MagParamsNoiseDensity=[ 0, 0, 0 ]  MagParamsBiasInstability=[ 0, 0, 0 ]  MagParamsBiasInstabilityNumerator=fractalcoef().Numerator  MagParamsBiasInstabilityDenominator=fractalcoef().Denominator  MagParamsRandomWalk=[ 0, 0, 0 ]  MagParamsNoiseType=double-sided  MagParamsTemperatureBias=[ 0, 0, 0 ]  MagParamsTemperatureScaleFactor=[ 0, 0, 0 ]
  PS-Simulink Converter : nesl_utility/PS-Simulink Converter  PhysicalDomain=network_engine_domain  SubClassName=ps_output  LeftPortType=input  RightPortType=output  PseudoPeriodic=off  Frequencies=[]  VectorFormat=inherit  Unit=rad  AffineConversion=off
  PS-Simulink Converter{1..3,7..9} (6 alike) : nesl_utility/PS-Simulink Converter  PhysicalDomain=network_engine_domain  SubClassName=ps_output  LeftPortType=input  RightPortType=output  PseudoPeriodic=off  Frequencies=[]  VectorFormat=inherit  Unit=rad/s  AffineConversion=off
  PS-Simulink Converter{4..6,10..12} (6 alike) : nesl_utility/PS-Simulink Converter  PhysicalDomain=network_engine_domain  SubClassName=ps_output  LeftPortType=input  RightPortType=output  PseudoPeriodic=off  Frequencies=[]  VectorFormat=inherit  Unit=m/s^2  AffineConversion=off
  Rate Transition : RateTransition  OutPortSampleTime=Fs_time
  Rate Transition1 : RateTransition  OutPortSampleTime=Fs_time
  Rate Transition2 : RateTransition  OutPortSampleTime=Fs_time
  Subtract1 : Sum
  Terminator{1..3,6} (4 alike) : Terminator
  Transpose : matrix_library/Transpose
  Vector Concatenate : Concatenate  NumInputs=3  Mode=Multidimensional array  ConcatenateDimension=2
  Vector Concatenate1 : Concatenate  NumInputs=3  Mode=Multidimensional array  ConcatenateDimension=2
  WorldFrame : PMIOPort  Side=Left
  SensorFrame : PMIOPort  Port=2  Side=Right
  Bus Element Out12 : Outport  PortName=GroundTruth  Element=wx
  Bus Element Out13 : Outport  PortName=GroundTruth  Element=wy
  Bus Element Out14 : Outport  PortName=GroundTruth  Element=wz
  Bus Element Out3 : Outport  PortName=GroundTruth  Element=ax
  Bus Element Out4 : Outport  PortName=GroundTruth  Element=ay
  Bus Element Out5 : Outport  PortName=GroundTruth  Element=az
  Bus Element Out6 : Outport  Port=2  PortName=Sensor1b  Element=wx
  Bus Element Out7 : Outport  Port=2  PortName=Sensor1b  Element=wy
  Bus Element Out8 : Outport  Port=2  PortName=Sensor1b  Element=wz
  Bus Element Out9 : Outport  Port=2  PortName=Sensor1b  Element=ax
  Bus Element Out10 : Outport  Port=2  PortName=Sensor1b  Element=ay
  Bus Element Out11 : Outport  Port=2  PortName=Sensor1b  Element=az
  Bus Element Out1 : Outport  Port=3  PortName=Sensor2b  Element=wx
  Bus Element Out2 : Outport  Port=3  PortName=Sensor2b  Element=wy
  Bus Element Out15 : Outport  Port=3  PortName=Sensor2b  Element=wz
  Bus Element Out16 : Outport  Port=3  PortName=Sensor2b  Element=ax
  Bus Element Out17 : Outport  Port=3  PortName=Sensor2b  Element=ay
  Bus Element Out18 : Outport  Port=3  PortName=Sensor2b  Element=az
  Bus Element Out19 : Outport  Port=4  PortName=Sensor3b  Element=wx
  Bus Element Out20 : Outport  Port=4  PortName=Sensor3b  Element=wy
  Bus Element Out21 : Outport  Port=4  PortName=Sensor3b  Element=wz
  Bus Element Out22 : Outport  Port=4  PortName=Sensor3b  Element=ax
  Bus Element Out23 : Outport  Port=4  PortName=Sensor3b  Element=ay
  Bus Element Out24 : Outport  Port=4  PortName=Sensor3b  Element=az
  Bus Element Out25 : Outport  Port=5  PortName=Sensor4b  Element=wx
  Bus Element Out26 : Outport  Port=5  PortName=Sensor4b  Element=wy
  Bus Element Out27 : Outport  Port=5  PortName=Sensor4b  Element=wz
  Bus Element Out28 : Outport  Port=5  PortName=Sensor4b  Element=ax
  Bus Element Out29 : Outport  Port=5  PortName=Sensor4b  Element=ay
  Bus Element Out30 : Outport  Port=5  PortName=Sensor4b  Element=az
  wires:
  Demux1/3 -> Bus Element Out8/1
  Demux1/2 -> Bus Element Out7/1
  Demux1/1 -> Bus Element Out6/1
  Constant1/1 -> Subtract1/2
  Rate Transition2/1 -> IMU 4b/3, IMU 3b/3, IMU 2b/3, IMU 1b/3
  Demux/2 -> Bus Element Out10/1
  Subtract1/1 -> Vector Concatenate/3
  Vector Concatenate/1 -> Rate Transition/1
  Rate Transition1/1 -> IMU 4b/2, IMU 3b/2, IMU 2b/2, IMU 1b/2
  IMU 1b/1 -> Demux/1
  IMU 1b/2 -> Demux1/1
  Demux/1 -> Bus Element Out9/1
  Demux/3 -> Bus Element Out11/1
  Transpose/1 -> Rate Transition2/1
  PS-Simulink Converter5/1 -> Vector Concatenate/2
  PS-Simulink Converter/1 -> Transpose/1
  Rate Transition/1 -> IMU 4b/1, IMU 3b/1, IMU 2b/1, IMU 1b/1
  Vector Concatenate1/1 -> Rate Transition1/1
  PS-Simulink Converter2/1 -> Vector Concatenate1/2
  PS-Simulink Converter1/1 -> Vector Concatenate1/1
  PS-Simulink Converter3/1 -> Vector Concatenate1/3
  PS-Simulink Converter6/1 -> Subtract1/1
  IMU 1b/3 -> Terminator6/1
  PS-Simulink Converter4/1 -> Vector Concatenate/1
  PS-Simulink Converter11/1 -> Gain1/1
  PS-Simulink Converter12/1 -> Gain2/1
  PS-Simulink Converter10/1 -> Gain/1
  PS-Simulink Converter9/1 -> Bus Element Out14/1
  PS-Simulink Converter8/1 -> Bus Element Out13/1
  PS-Simulink Converter7/1 -> Bus Element Out12/1
  Gain/1 -> Bus Element Out3/1
  Gain1/1 -> Bus Element Out4/1
  Gain2/1 -> Bus Element Out5/1
  Demux3/3 -> Bus Element Out15/1
  IMU 2b/1 -> Demux2/1
  Demux2/3 -> Bus Element Out18/1
  Demux2/2 -> Bus Element Out17/1
  Demux3/1 -> Bus Element Out1/1
  Demux3/2 -> Bus Element Out2/1
  Demux2/1 -> Bus Element Out16/1
  IMU 2b/2 -> Demux3/1
  IMU 2b/3 -> Terminator1/1
  Demux5/3 -> Bus Element Out21/1
  IMU 3b/1 -> Demux4/1
  Demux4/3 -> Bus Element Out24/1
  Demux4/2 -> Bus Element Out23/1
  Demux5/1 -> Bus Element Out19/1
  Demux5/2 -> Bus Element Out20/1
  Demux4/1 -> Bus Element Out22/1
  IMU 3b/2 -> Demux5/1
  IMU 3b/3 -> Terminator2/1
  Demux7/3 -> Bus Element Out27/1
  IMU 4b/1 -> Demux6/1
  Demux6/3 -> Bus Element Out30/1
  Demux6/2 -> Bus Element Out29/1
  Demux7/1 -> Bus Element Out25/1
  Demux7/2 -> Bus Element Out26/1
  Demux6/1 -> Bus Element Out28/1
  IMU 4b/2 -> Demux7/1
  IMU 4b/3 -> Terminator3/1
  connections:
  Generate input data for the IMU block/RConn6 -- PS-Simulink Converter4/LConn1
  PS-Simulink Converter1/LConn1 -- Generate input data for the IMU block/RConn3
  Generate input data for the IMU block/RConn7 -- PS-Simulink Converter5/LConn1
  Generate input data for the IMU block/RConn8 -- PS-Simulink Converter6/LConn1
  Generate input data for the IMU block/LConn1 -- Ground truth IMU data/LConn1 -- WorldFrame/RConn1
  Generate input data for the IMU block/RConn4 -- PS-Simulink Converter2/LConn1
  Generate input data for the IMU block/RConn5 -- PS-Simulink Converter3/LConn1
  PS-Simulink Converter/LConn1 -- Generate input data for the IMU block/RConn2
  SensorFrame/RConn1 -- Generate input data for the IMU block/RConn1 -- Ground truth IMU data/RConn1
  Ground truth IMU data/RConn2 -- PS-Simulink Converter7/LConn1
  Ground truth IMU data/RConn3 -- PS-Simulink Converter8/LConn1
  Ground truth IMU data/RConn5 -- PS-Simulink Converter10/LConn1
  Ground truth IMU data/RConn6 -- PS-Simulink Converter11/LConn1
  Ground truth IMU data/RConn7 -- PS-Simulink Converter12/LConn1
  Ground truth IMU data/RConn4 -- PS-Simulink Converter9/LConn1
